simulink model "ele2200_systemes"  (Simulink 8.1)
settings: Solver=ode45  StartTime=0.0  StopTime=1  RelTol=1e-3
settings Model: Creator=Administrateur  LastModifiedBy=ToniO
settings DataIOCC: SignalLoggingName=sigsOut
settings OptimizationCC: BooleanDataType=off  InitFltsAndDblsToZero=on
settings DebuggingCC: SaveWithParameterizedLinksMsg=none  SignalResolutionControl=TryResolveAllWithWarning  SolverPrmCheckMsg=none  MultiTaskDSMMsg=warning  MultiTaskCondExecSysMsg=none
settings HardwareCC: TargetUnknown=on
settings RTWCC: IncludeERTFirstTime=on
settings GRTTargetCC: TargetFcnLib=ansi_tfl_tmw.mat

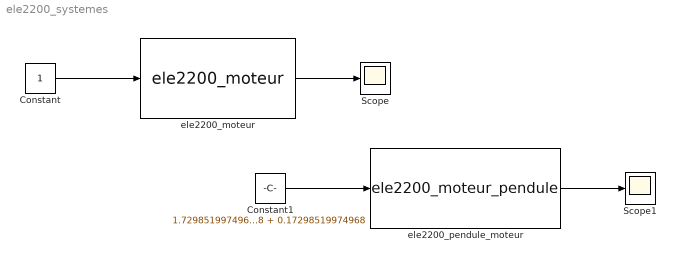
== system ele2200_systemes ==
  Constant : Constant
  Constant1 : Constant  Value=1.7298519974968 + 0.17298519974968
  Scope : Scope
  Scope1 : Scope
      settings: SaveName=theta
  ele2200_moteur : S-Function  FunctionName=ele2200_moteur  EnableBusSupport=off  mask(ele3200_labo3_mask){}
      mask Display:
      | patch([0 1.1 1.1 0 0], [1 1 -0.1 -0.1 1], [0.2 0.7 .5])
      | port_label('input', 1, '   u')
      | text(0.02, 0.5, '\n(Volts)', 'horizontalAlignment', 'left')
      | port_label('output', 1, ' w   ')
      | text(0.995, 0.5, '\n(rad/s)', 'horizontalAlignment', 'right')
      | text(0.35,0.55,'\n MOTEUR','horizontalAlignment')
  ele2200_pendule_moteur : S-Function  FunctionName=ele2200_moteur_pendule  Parameters=unit1,unit2  EnableBusSupport=off  mask(ele3200_labo3_mask){unit1=pi/5, unit2=1}
      mask prompts: unit1 "Position Angulaire Initiale"; unit2 "Courant Initial"
      mask Display:
      | patch([0 1.1 1.1 0 0], [1 1 -0.1 -0.1 1], [0 1 1])
      | port_label('input', 1, '   u')
      | text(0.02, 0.5, '\n(Volts)', 'horizontalAlignment', 'left')
      | port_label('output', 1, ' Theta  ')
      | text(0.995, 0.5, '\n(rad)   ', 'horizontalAlignment', 'right')
      | text(0.35,0.60,'\n MOTEUR','horizontalAlignment')
      | text(0.35,0.45,'\n + PENDULE','horizontalAlignment')
  wires:
  Constant/1 -> ele2200_moteur/1
  ele2200_moteur/1 -> Scope/1
  Constant1/1 -> ele2200_pendule_moteur/1
  ele2200_pendule_moteur/1 -> Scope1/1
